simulink library "library01"  (Simulink 6.3)
settings Model: LastModifiedBy=deissenb

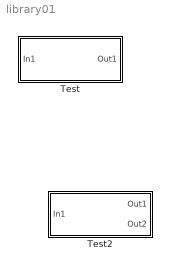
== system library01 ==
  Test : Subsystem
  Test2 : Subsystem

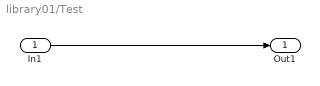
== system library01/Test ==
  In1 : Inport
  Out1 : Outport
  wires:
  In1/1 -> Out1/1

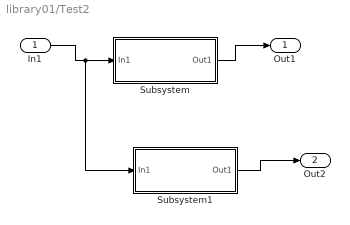
== system library01/Test2 ==
  In1 : Inport
  Subsystem : Subsystem
  Subsystem1 : Subsystem
  Out1 : Outport
  Out2 : Outport  Port=2
  wires:
  In1/1 -> Subsystem/1(In1), Subsystem1/1(In1)
  Subsystem/1(Out1) -> Out1/1
  Subsystem1/1(Out1) -> Out2/1

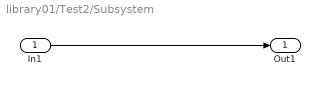
== system library01/Test2/Subsystem ==
  In1 : Inport
  Out1 : Outport
  wires:
  In1/1 -> Out1/1

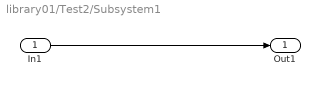
== system library01/Test2/Subsystem1 ==
  In1 : Inport
  Out1 : Outport
  wires:
  In1/1 -> Out1/1
